simulink model "simulation_upgrade"  (R2024b)
settings: Solver=ode1be  StartTime=0.0  StopTime=10  FixedStep=0.001  RelTol=1e-3
model workspace (MAT data in the model file):
  AMP = 1
  FREQ = 1
  i_abc = 1
values from neighbouring files (symbols this model uses):
  v_WLTP = [0 0 0 0 0 0 0 0 0 0 0 0 ... (180001 elements, 1x180001)]    [v_WLTP.mat]
undefined symbols (not defined in the file or in its folder): A, a_sig, b_sig, C1, C2, C3, Cd, CG_z, downshift, Drive_wheel, Driveshaft, f_blend, f_OVD, fo, front_seat_dist, fs, g, Gearbox, i, i_sig, Inclination, Inertia, Jr2, K, m, M_curve_1, M_curve_2, m_driver, M_N_1, M_N_2, mi_c, mi_s, Mode, N_clutch, n_curve_1, n_curve_2, n_driver, n_max_1, n_max_2, n_shift, n_surfaces, Pl, Planetary, r_eq_clutch, r_geom, r_wheel, rho, Shaft, shift_time, sigma0, sigma1, sigma2, slope_angle, Stage1, Stage2, Stage3, upshift, v0, vel_wind, vs ... (+5)
libraries: simulink x29, slpidlib x3
(part 9 of 9)

== system simulation_upgrade/DRIVETRAIN/Transmission/Gearbox/AMT/Clutch/Clutch1/Subsystem2 ==
  v : Inport
  z_dot : Inport  Port=2
  z : Inport  Port=3
  " " : Inport  Port=4
  Gain : Gain  Gain=sigma2
  Gain1 : Gain  Gain=sigma1
  Gain2 : Gain  Gain=sigma0
  Scope : Scope  NumInputPorts=3
  Sum3 : Sum  Inputs=+++
  Switch : Switch  Criteria=u2 ~= 0  SaturateOnIntegerOverflow=off  InputSameDT=off
  F : Outport
  wires:
  z/1 -> Gain2/1
  z_dot/1 -> Gain1/1
  Gain1/1 -> Sum3/2, Scope/2
  Sum3/1 -> Switch/1  "F"
  Gain2/1 -> Sum3/3, Scope/1
  Gain/1 -> Sum3/1, Scope/3
  v/1 -> Gain/1
  " "/1 -> Switch/2, Switch/3
  Switch/1 -> F/1

== system simulation_upgrade/DRIVETRAIN/Transmission/Gearbox/AMT/Stage_1/Spur/Shaft1 ==
  Torque_in : Inport
  Speed_fdbk : Inport  Port=2
  Derivative : Derivative
  Gain3 : Gain  Gain=J
  Sum1 : Sum  Inputs=|+-
  Torque_out : Outport
  phi_dot : Outport  Port=2
  wires:
  Sum1/1 -> Torque_out/1
  Torque_in/1 -> Sum1/1
  Speed_fdbk/1 -> phi_dot/1, Derivative/1
  Derivative/1 -> Gain3/1
  Gain3/1 -> Sum1/2

== system simulation_upgrade/DRIVETRAIN/Transmission/Gearbox/AMT/Stage_1/Spur/Spur1 ==
  Torque_in : Inport
  Speed_fdbk : Inport  Port=2
  Derivative : Derivative
  Derivative1 : Derivative
  Gain : Gain  Gain=i
  Gain2 : Gain  Gain=J2
  Gain3 : Gain  Gain=J1
  Gain4 : Gain  Gain=i
  Scope : Scope  NumInputPorts=2
  Sum1 : Sum  Inputs=|+-
  Sum2 : Sum  Inputs=|+-
  Torque_out : Outport
  phi_dot : Outport  Port=2
  wires:
  Gain/1 -> Sum2/1
  Sum2/1 -> Torque_out/1
  Torque_in/1 -> Sum1/1
  Gain4/1 -> Derivative1/1, phi_dot/1
  Speed_fdbk/1 -> Gain4/1, Derivative/1
  Sum1/1 -> Gain/1
  Derivative1/1 -> Gain3/1
  Derivative/1 -> Gain2/1
  Gain3/1 -> Scope/2, Sum1/2
  Gain2/1 -> Sum2/2, Scope/1

== system simulation_upgrade/DRIVETRAIN/Transmission/Gearbox/AMT/Stage_2.1/Spur/Spur2 ==
  Torque_in : Inport
  Speed_fdbk : Inport  Port=2
  Derivative1 : Derivative
  Gain : Gain  Gain=i
  Gain3 : Gain  Gain=J2
  Gain4 : Gain  Gain=i
  Sum1 : Sum  Inputs=|+-
  Torque_out : Outport
  phi_dot : Outport  Port=2
  wires:
  Sum1/1 -> Torque_out/1
  Gain3/1 -> Sum1/2
  Torque_in/1 -> Gain/1
  Speed_fdbk/1 -> Derivative1/1, Gain4/1
  Derivative1/1 -> Gain3/1
  Gain4/1 -> phi_dot/1
  Gain/1 -> Sum1/1

== system simulation_upgrade/DRIVETRAIN/Transmission/Gearbox/AMT/Stage_2.2/Spur/Spur2 ==
  Torque_in : Inport
  Speed_fdbk : Inport  Port=2
  Derivative1 : Derivative
  Gain : Gain  Gain=i
  Gain3 : Gain  Gain=J2
  Gain4 : Gain  Gain=i
  Sum1 : Sum  Inputs=|+-
  Torque_out : Outport
  phi_dot : Outport  Port=2
  wires:
  Sum1/1 -> Torque_out/1
  Torque_in/1 -> Gain/1
  Speed_fdbk/1 -> Derivative1/1, Gain4/1
  Derivative1/1 -> Gain3/1
  Gain3/1 -> Sum1/2
  Gain/1 -> Sum1/1
  Gain4/1 -> phi_dot/1

== system simulation_upgrade/DRIVETRAIN/Transmission/Gearbox/AMT/Stage_3/Spur/Shaft ==
  Torque_in : Inport
  Speed_fdbk : Inport  Port=2
  Derivative : Derivative
  Gain3 : Gain  Gain=J
  Sum1 : Sum  Inputs=|+-
  Torque_out : Outport
  phi_dot : Outport  Port=2
  wires:
  Speed_fdbk/1 -> phi_dot/1, Derivative/1
  Sum1/1 -> Torque_out/1
  Derivative/1 -> Gain3/1
  Torque_in/1 -> Sum1/1
  Gain3/1 -> Sum1/2

== system simulation_upgrade/DRIVETRAIN/Transmission/Gearbox/AMT/Stage_3/Spur/Spur3 ==
  Torque_in : Inport
  Speed_fdbk : Inport  Port=2
  Derivative : Derivative
  Derivative1 : Derivative
  Gain1 : Gain  Gain=i
  Gain2 : Gain  Gain=J2
  Gain3 : Gain  Gain=J1
  Gain5 : Gain  Gain=i
  Sum1 : Sum  Inputs=|+-
  Sum2 : Sum  Inputs=|+-
  Torque_out : Outport
  phi_dot : Outport  Port=2
  wires:
  Sum2/1 -> Torque_out/1
  Torque_in/1 -> Sum1/1
  Gain1/1 -> Sum2/1
  Sum1/1 -> Gain1/1
  Speed_fdbk/1 -> Gain5/1, Derivative/1
  Gain5/1 -> phi_dot/1, Derivative1/1
  Derivative/1 -> Gain2/1
  Derivative1/1 -> Gain3/1
  Gain3/1 -> Sum1/2
  Gain2/1 -> Sum2/2

== system simulation_upgrade/DRIVETRAIN/Transmission/Gearbox/AT/Stage_3/Spur/Spur3 ==
  Torque_in : Inport
  Speed_fdbk : Inport  Port=2
  Derivative : Derivative
  Derivative1 : Derivative
  Gain1 : Gain  Gain=i
  Gain2 : Gain  Gain=J2
  Gain3 : Gain  Gain=J1
  Gain5 : Gain  Gain=i
  Sum1 : Sum  Inputs=|+-
  Sum2 : Sum  Inputs=|+-
  Torque_out : Outport
  phi_dot : Outport  Port=2
  wires:
  Sum2/1 -> Torque_out/1
  Torque_in/1 -> Sum1/1
  Gain1/1 -> Sum2/1
  Sum1/1 -> Gain1/1
  Gain2/1 -> Sum2/2
  Gain3/1 -> Sum1/2
  Speed_fdbk/1 -> Gain5/1, Derivative/1
  Gain5/1 -> phi_dot/1, Derivative1/1
  Derivative/1 -> Gain2/1
  Derivative1/1 -> Gain3/1

== system simulation_upgrade/DRIVETRAIN/Transmission/Gearbox/DCT/Clutch1/Clutch1/Subsystem ==
  N : Inport
  v : Inport  Port=2
  Abs : Abs  SaturateOnIntegerOverflow=off
  Constant1 : Constant  Value=vs
  Divide1 : Product  Inputs=/*
  Divide2 : Product  Inputs=/*
  Exp : Math
  Gain1 : Gain  Gain=n_surfaces
  Gain4 : Gain  Gain=mi_s
  Gain5 : Gain  Gain=1/sigma0
  Gain6 : Gain  Gain=mi_c
  Gain7 : Gain  Gain=N_clutch*2
  Square : Math  Operator=square
  Sum4 : Sum  Inputs=+|+
  Sum5 : Sum  Inputs=|+-
  g(v) : Outport
  wires:
  Gain1/1 -> Gain4/1, Gain6/1
  Gain4/1 -> Sum5/1  "Fs"
  Abs/1 -> Gain7/1
  v/1 -> Divide1/2
  N/1 -> Abs/1
  Gain5/1 -> g(v)/1  "g(v)"
  Square/1 -> Exp/1
  Divide1/1 -> Square/1
  Constant1/1 -> Divide1/1
  Gain7/1 -> Gain1/1  "Fn"
  Exp/1 -> Divide2/1
  Gain6/1 -> Sum5/2, Sum4/2  "Fc"
  Divide2/1 -> Sum4/1
  Sum5/1 -> Divide2/2
  Sum4/1 -> Gain5/1

== system simulation_upgrade/DRIVETRAIN/Transmission/Gearbox/DCT/Clutch1/Clutch1/Subsystem1 ==
  v : Inport
  g(v) : Inport  Port=2
  " " : Inport  Port=3
  Abs1 : Abs  SaturateOnIntegerOverflow=off
  Compare To Zero1 : simulink/Logic and Bit Operations/Compare To Zero  relop=>  OutDataTypeStr=boolean
  Divide : Product  Inputs=*/
  Integrator : Integrator  ExternalReset=either
  Product : Product
  Product1 : Product
  Product2 : Product
  Saturation : Saturate  UpperLimit=inf  LowerLimit=0.01
  Sum2 : Sum  Inputs=|+-
  z_dot : Outport
  z : Outport  Port=2
  wires:
  Compare To Zero1/1 -> Integrator/2
  g(v)/1 -> Saturation/1
  Product2/1 -> Sum2/2
  Abs1/1 -> Divide/1
  Saturation/1 -> Divide/2
  Sum2/1 -> Integrator/1, Product1/1  "z_dot"
  v/1 -> Abs1/1, Sum2/1
  Divide/1 -> Product2/1
  Integrator/1 -> Product/2, Product2/2  "z"
  " "/1 -> Product1/2, Product/1, Compare To Zero1/1
  Product/1 -> z/1
  Product1/1 -> z_dot/1

== system simulation_upgrade/DRIVETRAIN/Transmission/Gearbox/DCT/Clutch1/Clutch1/Subsystem2 ==
  v : Inport
  z_dot : Inport  Port=2
  z : Inport  Port=3
  " " : Inport  Port=4
  Gain : Gain  Gain=sigma2
  Gain1 : Gain  Gain=sigma1
  Gain2 : Gain  Gain=sigma0
  Scope : Scope  NumInputPorts=3
  Sum3 : Sum  Inputs=+++
  Switch : Switch  Criteria=u2 > Threshold  Threshold=0.01  SaturateOnIntegerOverflow=off  InputSameDT=off
  F : Outport
  wires:
  z/1 -> Gain2/1
  z_dot/1 -> Gain1/1
  Gain1/1 -> Sum3/2, Scope/2
  Sum3/1 -> Switch/1  "F"
  Gain2/1 -> Sum3/3, Scope/1
  Gain/1 -> Sum3/1, Scope/3
  v/1 -> Gain/1
  " "/1 -> Switch/3, Switch/2
  Switch/1 -> F/1

== system simulation_upgrade/DRIVETRAIN/Transmission/Gearbox/DCT/Clutch1/Clutch2/Subsystem ==
  N : Inport
  v : Inport  Port=2
  Abs : Abs  SaturateOnIntegerOverflow=off
  Constant1 : Constant  Value=vs
  Divide1 : Product  Inputs=/*
  Divide2 : Product  Inputs=/*
  Exp : Math
  Gain1 : Gain  Gain=n_surfaces
  Gain4 : Gain  Gain=mi_s
  Gain5 : Gain  Gain=1/sigma0
  Gain6 : Gain  Gain=mi_c
  Gain7 : Gain  Gain=N_clutch*2
  Square : Math  Operator=square
  Sum4 : Sum  Inputs=+|+
  Sum5 : Sum  Inputs=|+-
  g(v) : Outport
  wires:
  Sum4/1 -> Gain5/1
  Sum5/1 -> Divide2/2
  Divide2/1 -> Sum4/1
  Gain6/1 -> Sum4/2, Sum5/2  "Fc"
  Exp/1 -> Divide2/1
  Gain7/1 -> Gain1/1  "Fn"
  Constant1/1 -> Divide1/1
  Divide1/1 -> Square/1
  Square/1 -> Exp/1
  Gain5/1 -> g(v)/1  "g(v)"
  N/1 -> Abs/1
  v/1 -> Divide1/2
  Abs/1 -> Gain7/1
  Gain4/1 -> Sum5/1  "Fs"
  Gain1/1 -> Gain6/1, Gain4/1

== system simulation_upgrade/DRIVETRAIN/Transmission/Gearbox/DCT/Clutch1/Clutch2/Subsystem1 ==
  v : Inport
  g(v) : Inport  Port=2
  " " : Inport  Port=3
  Abs1 : Abs  SaturateOnIntegerOverflow=off
  Compare To Zero1 : simulink/Logic and Bit Operations/Compare To Zero  relop=>  OutDataTypeStr=boolean
  Divide : Product  Inputs=*/
  Integrator : Integrator  ExternalReset=either
  Product : Product
  Product1 : Product
  Product2 : Product
  Saturation : Saturate  UpperLimit=inf  LowerLimit=0.01
  Sum2 : Sum  Inputs=|+-
  z_dot : Outport
  z : Outport  Port=2
  wires:
  Product1/1 -> z_dot/1
  Product/1 -> z/1
  " "/1 -> Compare To Zero1/1, Product/1, Product1/2
  Integrator/1 -> Product2/2, Product/2  "z"
  Divide/1 -> Product2/1
  v/1 -> Sum2/1, Abs1/1
  Sum2/1 -> Product1/1, Integrator/1  "z_dot"
  Saturation/1 -> Divide/2
  Abs1/1 -> Divide/1
  Product2/1 -> Sum2/2
  g(v)/1 -> Saturation/1
  Compare To Zero1/1 -> Integrator/2

== system simulation_upgrade/DRIVETRAIN/Transmission/Gearbox/DCT/Clutch1/Clutch2/Subsystem2 ==
  v : Inport
  z_dot : Inport  Port=2
  z : Inport  Port=3
  " " : Inport  Port=4
  Gain : Gain  Gain=sigma2
  Gain1 : Gain  Gain=sigma1
  Gain2 : Gain  Gain=sigma0
  Scope : Scope  NumInputPorts=3
  Sum3 : Sum  Inputs=+++
  Switch : Switch  Criteria=u2 > Threshold  Threshold=0.01  SaturateOnIntegerOverflow=off  InputSameDT=off
  F : Outport
  wires:
  Switch/1 -> F/1
  " "/1 -> Switch/2, Switch/3
  v/1 -> Gain/1
  Gain/1 -> Scope/3, Sum3/1
  Gain2/1 -> Scope/1, Sum3/3
  Sum3/1 -> Switch/1  "F"
  Gain1/1 -> Scope/2, Sum3/2
  z_dot/1 -> Gain1/1
  z/1 -> Gain2/1

== system simulation_upgrade/DRIVETRAIN/Transmission/Gearbox/DCT/Stage_2.1/Spur/Spur2 ==
  Torque_in : Inport
  Speed_fdbk : Inport  Port=2
  Derivative1 : Derivative
  Gain : Gain  Gain=i
  Gain3 : Gain  Gain=J2
  Gain4 : Gain  Gain=i
  Sum1 : Sum  Inputs=|+-
  Torque_out : Outport
  phi_dot : Outport  Port=2
  wires:
  Sum1/1 -> Torque_out/1
  Gain3/1 -> Sum1/2
  Torque_in/1 -> Gain/1
  Speed_fdbk/1 -> Derivative1/1, Gain4/1
  Derivative1/1 -> Gain3/1
  Gain4/1 -> phi_dot/1
  Gain/1 -> Sum1/1

== system simulation_upgrade/DRIVETRAIN/Transmission/Gearbox/DCT/Stage_2.2/Spur/Spur2 ==
  Torque_in : Inport
  Speed_fdbk : Inport  Port=2
  Derivative1 : Derivative
  Gain : Gain  Gain=i
  Gain3 : Gain  Gain=J2
  Gain4 : Gain  Gain=i
  Sum1 : Sum  Inputs=|+-
  Torque_out : Outport
  phi_dot : Outport  Port=2
  wires:
  Sum1/1 -> Torque_out/1
  Torque_in/1 -> Gain/1
  Speed_fdbk/1 -> Derivative1/1, Gain4/1
  Derivative1/1 -> Gain3/1
  Gain3/1 -> Sum1/2
  Gain/1 -> Sum1/1
  Gain4/1 -> phi_dot/1

== system simulation_upgrade/DRIVETRAIN/Transmission/Gearbox/DCT/Stage_3/Spur/Shaft ==
  Torque_in : Inport
  Speed_fdbk : Inport  Port=2
  Derivative : Derivative
  Gain3 : Gain  Gain=J
  Sum1 : Sum  Inputs=|+-
  Torque_out : Outport
  phi_dot : Outport  Port=2
  wires:
  Speed_fdbk/1 -> phi_dot/1, Derivative/1
  Sum1/1 -> Torque_out/1
  Derivative/1 -> Gain3/1
  Torque_in/1 -> Sum1/1
  Gain3/1 -> Sum1/2

== system simulation_upgrade/DRIVETRAIN/Transmission/Gearbox/DCT/Stage_3/Spur/Spur3 ==
  Torque_in : Inport
  Speed_fdbk : Inport  Port=2
  Derivative : Derivative
  Derivative1 : Derivative
  Gain1 : Gain  Gain=i
  Gain2 : Gain  Gain=J2
  Gain3 : Gain  Gain=J1
  Gain5 : Gain  Gain=i
  Sum1 : Sum  Inputs=|+-
  Sum2 : Sum  Inputs=|+-
  Torque_out : Outport
  phi_dot : Outport  Port=2
  wires:
  Sum2/1 -> Torque_out/1
  Torque_in/1 -> Sum1/1
  Gain1/1 -> Sum2/1
  Sum1/1 -> Gain1/1
  Speed_fdbk/1 -> Gain5/1, Derivative/1
  Gain5/1 -> phi_dot/1, Derivative1/1
  Derivative/1 -> Gain2/1
  Derivative1/1 -> Gain3/1
  Gain3/1 -> Sum1/2
  Gain2/1 -> Sum2/2

== system simulation_upgrade/DRIVETRAIN/Transmission/Gearbox/TDT/Stage_1/Spur/Shaft1 ==
  Torque_in : Inport
  Speed_fdbk : Inport  Port=2
  Derivative : Derivative
  Gain3 : Gain  Gain=J
  Sum1 : Sum  Inputs=|+-
  Torque_out : Outport
  phi_dot : Outport  Port=2
  wires:
  Sum1/1 -> Torque_out/1
  Gain3/1 -> Sum1/2
  Torque_in/1 -> Sum1/1
  Speed_fdbk/1 -> phi_dot/1, Derivative/1
  Derivative/1 -> Gain3/1

== system simulation_upgrade/DRIVETRAIN/Transmission/Gearbox/TDT/Stage_1/Spur/Spur1 ==
  Torque_in : Inport
  Speed_fdbk : Inport  Port=2
  Derivative : Derivative
  Derivative1 : Derivative
  Gain : Gain  Gain=i
  Gain2 : Gain  Gain=J2
  Gain3 : Gain  Gain=J1
  Gain4 : Gain  Gain=i
  Sum1 : Sum  Inputs=|+-
  Sum2 : Sum  Inputs=|+-
  Torque_out : Outport
  phi_dot : Outport  Port=2
  wires:
  Gain/1 -> Sum2/1
  Sum2/1 -> Torque_out/1
  Gain3/1 -> Sum1/2
  Torque_in/1 -> Sum1/1
  Gain4/1 -> Derivative1/1, phi_dot/1
  Speed_fdbk/1 -> Gain4/1, Derivative/1
  Gain2/1 -> Sum2/2
  Sum1/1 -> Gain/1
  Derivative1/1 -> Gain3/1
  Derivative/1 -> Gain2/1

== system simulation_upgrade/DRIVETRAIN/Transmission/Gearbox/TDT/Stage_2.1/Spur/Shaft1 ==
  Torque_in : Inport
  Speed_fdbk : Inport  Port=2
  Derivative : Derivative
  Gain3 : Gain  Gain=J
  Sum1 : Sum  Inputs=|+-
  Torque_out : Outport
  phi_dot : Outport  Port=2
  wires:
  Speed_fdbk/1 -> phi_dot/1, Derivative/1
  Sum1/1 -> Torque_out/1
  Derivative/1 -> Gain3/1
  Gain3/1 -> Sum1/2
  Torque_in/1 -> Sum1/1

== system simulation_upgrade/DRIVETRAIN/Transmission/Gearbox/TDT/Stage_2.1/Spur/Spur2 ==
  Torque_in : Inport
  Speed_fdbk : Inport  Port=2
  Derivative : Derivative
  Derivative1 : Derivative
  Gain : Gain  Gain=i
  Gain2 : Gain  Gain=J2
  Gain3 : Gain  Gain=J1
  Gain4 : Gain  Gain=i
  Sum1 : Sum  Inputs=|+-
  Sum2 : Sum  Inputs=|+-
  Torque_out : Outport
  phi_dot : Outport  Port=2
  wires:
  Gain/1 -> Sum2/1
  Sum2/1 -> Torque_out/1
  Gain3/1 -> Sum1/2
  Torque_in/1 -> Sum1/1
  Gain4/1 -> Derivative1/1, phi_dot/1
  Speed_fdbk/1 -> Gain4/1, Derivative/1
  Gain2/1 -> Sum2/2
  Sum1/1 -> Gain/1
  Derivative1/1 -> Gain3/1
  Derivative/1 -> Gain2/1

== system simulation_upgrade/DRIVETRAIN/Transmission/Gearbox/TDT/Stage_2.2/Spur/Shaft1 ==
  Torque_in : Inport
  Speed_fdbk : Inport  Port=2
  Derivative : Derivative
  Gain3 : Gain  Gain=J
  Sum1 : Sum  Inputs=|+-
  Torque_out : Outport
  phi_dot : Outport  Port=2
  wires:
  Speed_fdbk/1 -> phi_dot/1, Derivative/1
  Sum1/1 -> Torque_out/1
  Derivative/1 -> Gain3/1
  Gain3/1 -> Sum1/2
  Torque_in/1 -> Sum1/1

== system simulation_upgrade/DRIVETRAIN/Transmission/Gearbox/TDT/Stage_2.2/Spur/Spur2 ==
  Torque_in : Inport
  Speed_fdbk : Inport  Port=2
  Derivative : Derivative
  Derivative1 : Derivative
  Gain : Gain  Gain=i
  Gain2 : Gain  Gain=J2
  Gain3 : Gain  Gain=J1
  Gain4 : Gain  Gain=i
  Sum1 : Sum  Inputs=|+-
  Sum2 : Sum  Inputs=|+-
  Torque_out : Outport
  phi_dot : Outport  Port=2
  wires:
  Gain/1 -> Sum2/1
  Sum2/1 -> Torque_out/1
  Gain3/1 -> Sum1/2
  Torque_in/1 -> Sum1/1
  Gain4/1 -> Derivative1/1, phi_dot/1
  Speed_fdbk/1 -> Gain4/1, Derivative/1
  Gain2/1 -> Sum2/2
  Sum1/1 -> Gain/1
  Derivative1/1 -> Gain3/1
  Derivative/1 -> Gain2/1

== system simulation_upgrade/DRIVETRAIN/Transmission/Gearbox/TDT/Stage_3/Spur/Spur3 ==
  Torque_in : Inport
  Speed_fdbk : Inport  Port=2
  Derivative : Derivative
  Derivative1 : Derivative
  Gain : Gain  Gain=i
  Gain2 : Gain  Gain=J2
  Gain3 : Gain  Gain=J1
  Gain4 : Gain  Gain=i
  Sum1 : Sum  Inputs=|+-
  Sum2 : Sum  Inputs=|+-
  Torque_out : Outport
  phi_dot : Outport  Port=2
  wires:
  Gain/1 -> Sum2/1
  Sum2/1 -> Torque_out/1
  Gain3/1 -> Sum1/2
  Torque_in/1 -> Sum1/1
  Gain4/1 -> Derivative1/1, phi_dot/1
  Speed_fdbk/1 -> Gain4/1, Derivative/1
  Gain2/1 -> Sum2/2
  Sum1/1 -> Gain/1
  Derivative1/1 -> Gain3/1
  Derivative/1 -> Gain2/1

== stateflow chart simulation_upgrade/CONTROLS/Main Control Unit/TDT_MCU/TDT_MCU ==
  state SteadyState_G2
    entry:
    shifting_stage = 0;
    C2_set = 2;
    during:
    M_MCU1 = M_EM1_Driver;
    M_MCU2 = M_EM2_Driver;
    exit:
    M_shift1 = M_MCU1;
    M_shift2 = M_MCU2;
  state Taking_off
    entry:
    Take_off = 1;
    C2_set = 1;
    during:
    M_MCU1 = M_EM1_Driver;
    M_MCU2 = M_EM2_Driver;
    exit:
    Take_off = 0;
  state TorqueBlend_PH1
    entry:
    shifting_stage = 1;
    during:
    M_MCU1 = M_MCU1 + f_blend/i_TG2 * 0.001;
    M_MCU2 = M_MCU2 - f_blend/i_TG1 *  0.001;
    M_MCU1 = max(min(M_MCU1, f_OVD*M_N_1), 0);
    M_MCU2 = max(min(M_MCU2, M_N_2), 0);
  state TorqueBlend_PH7
    entry:
    shifting_stage = 7;
    during:
    M_MCU1 = M_MCU1 - f_blend/i_TG2 * 0.001;
    M_MCU1 = max(min(M_MCU1, f_OVD*M_N_1), M_shift1);
    if M_shift2 > M_MCU2
    M_MCU2 = M_MCU2 + f_blend/i_TG1 * 0.001;
    else
    M_MCU2 = M_MCU2 - f_blend/i_TG1 * 0.001;
    end
  state SteadyState_G1
    entry:
    shifting_stage = 0;
    C2_set = 1;
    during:
    M_MCU1 = M_EM1_Driver;
    M_MCU2 = M_EM2_Driver;
    exit:
    M_shift1 = M_MCU1;
    M_shift2 = M_MCU2;
  state TorqueBlend_PH2
    entry:
    shifting_stage = 2;
    during:
    M_MCU1 = M_MCU1;
    M_MCU2 = M_MCU2 - f_blend/i_TG1 *  0.001;
    M_MCU2 = max(min(M_MCU2, M_N_2), 0);
  state TorqueBlend_PH6
    entry:
    shifting_stage = 6;
    during:
    M_MCU1 = M_MCU1;
    M_MCU2 = M_MCU2 + f_blend/i_TG1 * 0.001;
    M_MCU2 = max(min(M_MCU2, M_shift2), -M_N_2);
  state Synch_PH4
    entry:
    shifting_stage = 4;
    during:
    M_MCU1 = M_MCU1;
    if GearSet == 1
    M_MCU2 = w_clutch - w_spur12;
    elseif GearSet == 2
    M_MCU2 = w_clutch - w_spur22;
    end
  state NeutralStage_PH3
    entry:
    shifting_stage = 3;
    C2_set = 0;
    during:
    M_MCU1 = M_MCU1;
    M_MCU2 = 0;
  state UpDownshift_PH5
    entry:
    shifting_stage = 5;
    C2_set = GearSet;
    during:
    M_MCU1 = M_MCU1;
    M_MCU2 = 0;
  SteadyState_G2 -> TorqueBlend_PH1 [order 2] : [C2 >= 2 && n_engine<n_shift-3000 && Pedal>0 || downshift>0]{GearSet = 1}
  TorqueBlend_PH7 -> SteadyState_G2 [order 2] : [M_MCU1 == M_shift1 && M_MCU2 >= 0.99*M_shift2 && GearSet == 2]
  SteadyState_G2 -> Taking_off [order 1] : [w_clutch == 0]
  (default) -> Taking_off
  Taking_off -> SteadyState_G1 : [n_engine >= 100]
  SteadyState_G1 -> Taking_off [order 2] : [w_clutch == 0]
  SteadyState_G1 -> TorqueBlend_PH1 [order 1] : [C2==1 && shifting_stage==0 && n_engine>=n_shift & Pedal>0 || upshift>0 ]
      | {GearSet = 2}
  TorqueBlend_PH7 -> SteadyState_G1 [order 1] : [M_MCU1 <= M_shift1 && M_MCU2 >= M_shift2 && GearSet == 1]
  TorqueBlend_PH1 -> NeutralStage_PH3 [order 2] : [M_EM2 <= 0.01]
  TorqueBlend_PH1 -> TorqueBlend_PH2 [order 1] : [round(M_MCU1) == M_shift1*f_OVD]
  TorqueBlend_PH6 -> TorqueBlend_PH7 : [M_MCU2 >= M_shift2 - (M_MCU1-M_shift1)*i_TG2/i_TG1]
  TorqueBlend_PH2 -> NeutralStage_PH3 : [M_EM2 <= 0.01]
  UpDownshift_PH5 -> TorqueBlend_PH6 : [C2 >= 0.99*C2_set]
  NeutralStage_PH3 -> Synch_PH4 : [C2 <= 0 ]
  Synch_PH4 -> UpDownshift_PH5 : [w_clutch >= w_spur22 && GearSet == 2 || w_clutch <= w_spur12 && GearSet == 1]
  data: M_MCU1 output; M_MCU2 output; M_N_2 input; M_EM2 input; shifting_stage output =0; i_TG1 input; i_TG2 input; downshift input; n_engine input; n_shift input; upshift input; M_N_1 input; M_EM1_Driver input; M_EM2_Driver input; Pedal input; C2_set output =1; C2 input; w_clutch input; f_OVD input; w_spur12 input; w_spur22 input; acc input; f_blend input; Take_off output =0; GearSet output double =1; M_shift2 local; M_shift1 local

== stateflow chart simulation_upgrade/PANEL/Main Control Unit/Chart ==
  state Steady_State_G1
  state Taking_Off
  state Torque_Blend_PH1
  state Torque_Blend_PH7
  state Steady_State_G2
  state Torque_Blend_PH2
  state Torque_Blend_PH6
  state Neutral_Stage_PH3
  state Synch_PH4
  state UpDownshift_PH5
  state15 -> state18 [order 1] : [n_engine > n_ushift]
  state35 -> state15 [order 2] : [GearSet==1]
  state15 -> state5 [order 2] : [Speed == 0]
  state5 -> state15 : [n_engine > 100]
  (default) -> state5
  state20 -> state5 [order 2] : [Speed == 0]
  state20 -> state18 [order 1] : [n_engine < n_dshift]
  state35 -> state20 [order 1] : [GearSet == 2]
  state18 -> state19
  state33 -> state35
  state19 -> state24
  state31 -> state33
  state24 -> state26
  state26 -> state31
  data: output; input; input; output

== stateflow chart simulation_upgrade/CONTROLS/Main Control Unit/AT_MCU/AT_MCU ==
  state Taking_off
    entry:
    C2_set = 1;
    Take_off = 1;
    during:
    M_MCU1 = M_Driver;
    clutch2set = 1;
    exit:
    Take_off = 0;
  state SteadyState_G1
    entry:
    shifting_stage = 0;
    during:
    M_MCU1 = M_Driver;
    C2_set = 1;
    exit:
    GearSet = 2;
  state Upshifting
    entry:
    shifting_stage = 1;
    clutch1set = 1;
    clutch2set = 0;
  state Downshifting
    entry:
    shifting_stage = 1;
    clutch1set = 0;
    clutch2set = 1;
  state SteadyState_G2
    entry:
    shifting_stage = 0;
    C2_set = 2;
    during:
    M_MCU1 = M_Driver;
    exit:
    GearSet = 1;
  (default) -> Taking_off
  Taking_off -> SteadyState_G1 : [n_engine>=100]
  SteadyState_G1 -> Taking_off [order 2] : [Speed==0]
  Downshifting -> SteadyState_G1 : [clutch2 >= 0.99*clutch2set && clutch1 <= 0.01*clutch1set]
  SteadyState_G1 -> Upshifting [order 1] : [C2==1 && shifting_stage==0 && n_engine>=n_shift || upshift>0]
  Upshifting -> SteadyState_G2 : [clutch1 >= 0.99*clutch1set && clutch2 <= 0.01*clutch2set]
  SteadyState_G2 -> Downshifting : [C2 == 2 && n_engine<2000 && acc<0 || downshift>0]
  data: M_MCU1 output; shifting_stage output =0; Take_off output; C2_set output =1; upshift input; downshift input; n_engine input; Speed input; acc input; C2 input; M_Driver input; GearSet output size=1 =0; clutch2 input; clutch1 input; clutch2set output =0; clutch1set output =0; n_shift input

== stateflow chart simulation_upgrade/CONTROLS/Main Control Unit/DCT_MCU/DCT_MCU ==
  state SteadyState_G2
    entry:
    shifting_stage = 0;
    C2_set = 2;
    during:
    M_MCU = M_EM_Driver;
    exit:
    M_shift = M_MCU;
  state Inertia_phase
    entry:
    shifting_stage = 2;
    Take_off = 2;
    during:
    M_MCU = M_shift + wt2;
  state Taking_off
    entry:
    Take_off = 1;
    clutch1Set = 1;
    clutch2Set = 0;
    during:
    if M_EM_Driver > 0
    M_MCU = M_MCU + f_blend * 0.001;
    else
    M_MCU = 0;
    end
    exit:
    Take_off = 0;
  state Torque_phase
    entry:
    shifting_stage = 1;
    clutch1Set = 0;
    during:
    c2 = round((M_csum - M_c1*i1)/(i2*M_c2));
    M_MCU = M_shift;
  state SteadyState_G1
    entry:
    shifting_stage = 0;
    C2_set = 1;
    during:
    M_MCU = M_EM_Driver;
    exit:
    M_shift = M_MCU;
  Inertia_phase -> SteadyState_G2 : [wt2 == 0]
  SteadyState_G2 -> Taking_off : [n_engine == 0]
  Torque_phase -> Inertia_phase : [ M_c1 <= 1]
  (default) -> Taking_off
  Taking_off -> SteadyState_G1 : [n_engine >= 100 &&  abs(M_MCU) >= abs(M_EM_Driver)]
  SteadyState_G1 -> Taking_off [order 2] : [n_engine == 0]
  SteadyState_G1 -> Torque_phase [order 1] : [C2==1 && shifting_stage==0 && w_spur11>=w_clutch_upshift & Pedal>0]{GearSet = 2}
  data: M_MCU output =0; n_engine input; M_EM_Driver input; C2_set output =1; C2 input; i2 input; i1 input; M_c1 input; M_c2 input; M_csum input; Pedal input; Take_off output =0; shifting_stage output; c1 output =1; clutch1Set output =1; clutch2Set output =0; c2 output =0; GearSet output int32 =1; w_clutch_upshift input; wt1 input; wt2 input; w_engine input; M_shift local; f_blend input; we local; w_spur21 input; w_spur11 input

== stateflow chart simulation_upgrade/CONTROLS/Main Control Unit/AMT_MCU/AMT_MCU ==
  state SteadyState_G2
    entry:
    shifting_stage = 0;
    C2_set = 2;
    during:
    M_MCU = M_EM_Driver;
    exit:
    M_shift = M_MCU;
  state Taking_off
    entry:
    Take_off = 1;
    clutchSet = 1;
    during:
    if M_EM_Driver > 0
    M_MCU = M_MCU + f_blend * 0.001/2;
    else
    M_MCU = 0;
    end
    exit:
    Take_off = 0;
  state TorqueBlend_PH1
    entry:
    shifting_stage = 1;
    during:
    M_MCU = M_MCU - f_blend * 0.001;
  state TorqueBlend_PH5
    entry:
    shifting_stage = 5;
    during:
    M_MCU = M_MCU + f_blend * 0.001;
  state SteadyState_G1
    entry:
    shifting_stage = 0;
    C2_set = 1;
    during:
    M_MCU = M_EM_Driver;
    exit:
    M_shift = M_MCU;
  state ShiftingStage_PH4
    entry:
    shifting_stage = 4;
    C2_set = GearSet;
    if GearSet == 2
    clutchSet = -1;
    else
    clutchSet = 1;
    end
    during:
    M_MCU = 0;
  state Synch_PH3
    entry:
    shifting_stage = 3;
    C2_set = 0;
    during:
    if GearSet == 1
    M_MCU = w_clutch - w_spur11;
    elseif GearSet == 2
    M_MCU = -(w_clutch - w_spur21)/4
    end
  state DecoupleStage_PH2
    entry:
    shifting_stage = 2;
    clutchSet = 0;
    during:
    M_MCU = 0;
  TorqueBlend_PH5 -> SteadyState_G2 [order 2] : [M_MCU >= 0.99*M_shift  && GearSet == 2]
  SteadyState_G2 -> TorqueBlend_PH1 [order 1] : [C2 >= 2 && w_clutch<w_clutch_upshift-150 && Pedal>0 || downshift>0]{GearSet = 1}
  SteadyState_G2 -> Taking_off [order 2] : [w_clutch == 0]
  (default) -> Taking_off
  Taking_off -> SteadyState_G1 : [n_engine >= 100 &&  abs(M_MCU) >= abs(M_EM_Driver)]
  SteadyState_G1 -> Taking_off [order 1] : [w_clutch == 0]
  SteadyState_G1 -> TorqueBlend_PH1 [order 2] : [C2==1 && shifting_stage==0 && w_clutch>=w_clutch_upshift & Pedal>0 || upshift>0 ]{GearSet = 2}
  TorqueBlend_PH5 -> SteadyState_G1 [order 1] : [M_MCU >= 0.99*M_shift  && GearSet == 1]
  TorqueBlend_PH1 -> DecoupleStage_PH2 : [M_MCU <= 0]
  ShiftingStage_PH4 -> TorqueBlend_PH5 : [clutch == clutchSet]
  Synch_PH3 -> ShiftingStage_PH4 : [abs(w_clutch-w_spur21) <= 0.1 && GearSet == 2 || w_clutch >= w_spur11 && GearSet == 1]
  DecoupleStage_PH2 -> Synch_PH3 : [clutch == clutchSet]
  data: M_MCU output =0; shifting_stage output =0; downshift input; n_engine input; upshift input; M_EM_Driver input; C2_set output =1; C2 input; clutch input; w_clutch input; Pedal input; w_spur11 input; w_spur21 input; Take_off output =0; clutchSet output =1; GearSet output double =1; w_clutch_upshift input; f_blend input; M_shift local

== stateflow chart simulation_upgrade/CONTROLS/Main Control Unit/CVT_MCU/CVT_MCU ==
  state Taking_off
    entry:
    Take_off = 1;
    C2_set = 1;
    during:
    M_MCU1 = M_EM1_Driver;
    M_MCU2 = M_EM2_Driver;
    exit:
    Take_off = 0
  state SteadyState_G1
    entry:
    shifting_stage = 0;
    C2_set = 1;
    during:
    M_MCU1 = M_EM1_Driver;
    M_MCU2 = M_EM2_Driver;
  state NeutralStage_PH3
    entry:
    shifting_stage = 3;
    C2_set = 0;
    during:
    M_MCU1 = M_MCU1;
    M_MCU2 = 0;
  state Synch_PH4
    entry:
    shifting_stage = 4;
    during:
    M_MCU1 = M_MCU1;
    if GearSet == 1
    M_MCU2 = w_spur12 - w_clutch;
    elseif GearSet == 2
    M_MCU2 = w_clutch - w_spur22;
    end
  state UpDownshift_PH5
    entry:
    shifting_stage = 5;
    C2_set = GearSet;
    during:
    M_MCU1 = M_MCU1;
    M_MCU2 = 0;
  state TorqueBlend_PH6
    entry:
    shifting_stage = 6;
    during:
    M_MCU1 = M_MCU1;
    M_MCU2 = M_MCU2 + f_blend/i_TG1 * 0.001;
    M_MCU2 = max(min(M_MCU2, M_EM2_Driver), 0);
  state TorqueBlend_PH7
    entry:
    shifting_stage = 7;
    during:
    M_MCU1 = M_MCU1 - f_blend/i_TG2 * 0.001;
    M_MCU2 = M_MCU2 + f_blend/i_TG1 * 0.001;
    M_MCU1 = max(min(M_MCU1, f_OVD*M_N_1), M_EM1_Driver);
    M_MCU2 = max(min(M_MCU2, M_EM2_Driver), 0);
  state TorqueBlend_PH1
    entry:
    shifting_stage = 1;
    during:
    M_MCU1 = M_MCU1 + f_blend/i_TG2 * 0.001;
    M_MCU2 = M_MCU2 - f_blend/i_TG1 *  0.001;
    M_MCU1 = max(min(M_MCU1, f_OVD*M_N_1), -M_N_1);
    M_MCU2 = max(min(M_MCU2, M_N_2), 0);
  state TorqueBlend_PH2
    entry:
    shifting_stage = 2;
    during:
    M_MCU1 = M_MCU1;
    M_MCU2 = M_MCU2 - f_blend/i_TG1 *  0.001;
    M_MCU2 = max(min(M_MCU2, M_N_2), 0);
  state SteadyState_G2
    entry:
    shifting_stage = 0;
    C2_set = 2;
    during:
    M_MCU1 = M_EM1_Driver;
    M_MCU2 = M_EM2_Driver;
  (default) -> Taking_off
  Taking_off -> SteadyState_G1 : [n_engine >= 100]
  SteadyState_G1 -> Taking_off [order 2] : [w_clutch == 0]
  SteadyState_G1 -> TorqueBlend_PH1 [order 1] : [C2==1 && shifting_stage==0 && n_engine>=n_shift || upshift>0 ]{GearSet = 2}
  TorqueBlend_PH7 -> SteadyState_G1 [order 1] : [M_MCU1 <= 1.01*M_EM1_Driver && M_MCU2 >= 0.99*M_EM2_Driver && GearSet == 1]
  UpDownshift_PH5 -> TorqueBlend_PH6 : [C2 >= 0.99*C2_set]
  Synch_PH4 -> UpDownshift_PH5 : [w_clutch >= w_spur22 && GearSet == 2 || w_clutch <= w_spur12 && GearSet == 1]
  TorqueBlend_PH2 -> NeutralStage_PH3 : [M_EM2 <= 0.01]
  TorqueBlend_PH1 -> TorqueBlend_PH2 [order 1] : [round(M_MCU1) == M_EM1_Driver*f_OVD]
  NeutralStage_PH3 -> Synch_PH4 : [C2 <= 0 ]
  TorqueBlend_PH6 -> TorqueBlend_PH7 : [M_MCU2 >= M_EM2_Driver - (M_MCU1-M_EM1_Driver)*i_TG2/i_TG1]
  SteadyState_G2 -> TorqueBlend_PH1 : [C2 >= 2 && n_engine<2000 && acc<0 || downshift>0]{GearSet = 1}
  TorqueBlend_PH1 -> NeutralStage_PH3 [order 2] : [M_EM2 <= 0.01]
  TorqueBlend_PH7 -> SteadyState_G2 [order 2] : [M_MCU1 <= 1.01*M_EM1_Driver && M_MCU2 >= 0.99*M_EM2_Driver && GearSet == 2]
  data: M_MCU1 output; M_MCU2 output; M_N_2 input; M_EM2 input; shifting_stage output =0; i_TG1 input; i_TG2 input; downshift input; n_engine input; n_shift input; upshift input; M_N_1 input; M_EM1_Driver input; M_EM2_Driver input; C2_set output =1; C2 input; w_clutch input; f_OVD input; w_spur12 input; w_spur22 input; acc input; f_blend input; Take_off output =0; GearSet output double =1

== stateflow chart simulation_upgrade/PANEL/Pretty shot/Main Control Unit /Chart ==
  state Steady_State_G1
  state Taking_Off
  state Torque_Blend_PH1
  state Torque_Blend_PH7
  state Steady_State_G2
  state Torque_Blend_PH2
  state Torque_Blend_PH6
  state Neutral_Stage_PH3
  state Synch_PH4
  state UpDownshift_PH5
  state15 -> state18 [order 1] : [n_engine > n_shift]
  state35 -> state15 [order 2] : [GearSet==1]
  state15 -> state5 [order 2] : [Speed == 0]
  state5 -> state15 : [n_engine > 100]
  (default) -> state5
  state20 -> state5 [order 2] : [Speed == 0]
  state20 -> state18 [order 1] : [n_engine < 2000]
  state35 -> state20 [order 1] : [GearSet == 2]
  state18 -> state19
  state33 -> state35
  state19 -> state24
  state31 -> state33
  state24 -> state26
  state26 -> state31
  data: output; input; input; output
